simulink model "control_pid_nolineal"  (R2022b)
settings: Solver=ode45  StartTime=0.0  StopTime=30  MaxStep=0.01  RelTol=1e-3  EnableMultiTasking=on
values from neighbouring files (symbols this model uses):
  A = XX    [codigo_Prac5.m]
  k = As*sqrt(2*g)    [codigo_Prac5.m]
  Kp = XX    [codigo_Prac5.m]
  Q = 2    [codigo_Prac5.m]
  Td = XX    [codigo_Prac5.m]
  Ti = XX    [codigo_Prac5.m]
  x0_ini = [2*XX  XX]    [codigo_Prac5.m]
settings Model: Creator=carles  LastModifiedBy=ggarc
settings SolverCC: AlgebraicLoopSolver=TrustRegion
settings DataIOCC: LimitDataPoints=on  SaveFormat=Array  SignalLoggingSaveFormat=ModelDataLogs  ReturnWorkspaceOutputs=off
settings OptimizationCC: ExpressionDepthLimit=2147483647  LifeSpan=inf
settings DebuggingCC: UnderspecifiedInitializationDetection=Classic  MergeDetectMultiDrivingBlocksExec=none  SolverPrmCheckMsg=warning  FcnCallInpInsideContextMsg=warning  UnconnectedInputMsg=warning  UnconnectedOutputMsg=warning  UnconnectedLineMsg=warning  StateNameClashWarn=warning  SFUnexpectedBacktrackingDiag=warning  SFNoUnconditionalDefaultTransitionDiag=warning  SFExecutionAtInitializationDiag=none  SFMachineParentedDataDiag=warning  ArithmeticOperatorsInVariantConditions=warning
settings HardwareCC: ProdBitPerPointer=32  ProdBitPerSizeT=32  ProdBitPerPtrDiffT=32  ProdLargestAtomicFloat=None  ProdIntDivRoundTo=Undefined  ProdEndianess=Unspecified  ProdWordSize=32  ProdHWDeviceType=32-bit Generic
settings ModelReferenceCC: PropagateSignalLabelsOutOfModel=off
settings SFSimCC: SimUseLocalCustomCode=off  CustomCodeUndefinedFunction=UseInterfaceOnly
settings RTWCC: RTWUseLocalCustomCode=off
settings CodeAppCC: StateflowObjectComments=on
settings GRTTargetCC: TargetLangStandard=C89/C90 (ANSI)  CombineOutputUpdateFcns=off  GRTInterface=on
settings ConfigComp: CovMetricSettings=dw  CovSaveCumulativeToWorkspaceVar=on  CovSaveSingleToWorkspaceVar=on  CovExternalEMLEnable=off  CovSFcnEnable=off

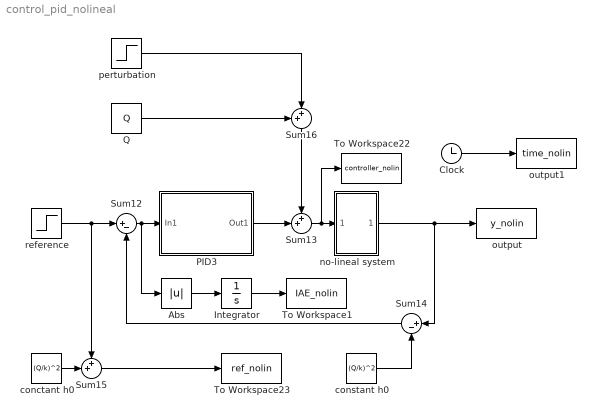
== system control_pid_nolineal ==
  Abs : Abs  SaturateOnIntegerOverflow=off
  Clock : Clock
  Integrator : Integrator
  PID3 : Subsystem
  Q : Constant  Value=Q
  Sum12 : Sum  Inputs=|+-
  Sum13 : Sum  Inputs=++|
  Sum14 : Sum  Inputs=|+-
  Sum15 : Sum  Inputs=++|
  Sum16 : Sum  Inputs=++|
  To Workspace1 : ToWorkspace  VariableName=IAE_nolin  SampleTime=-1
  To Workspace22 : ToWorkspace  VariableName=controller_nolin  SaveFormat=Structure With Time  SampleTime=-1
  To Workspace23 : ToWorkspace  VariableName=ref_nolin  SaveFormat=Structure With Time  SampleTime=-1
  conctant h0 : Constant  Value=(Q/k)^2
  constant h0 : Constant  Value=(Q/k)^2
  no-lineal system : Subsystem
  output : ToWorkspace  VariableName=y_nolin  SaveFormat=Structure With Time  SampleTime=-1
  output1 : ToWorkspace  VariableName=time_nolin  SampleTime=-1
  perturbation : Step  Time=30  After=2  SampleTime=0
  reference : Step  Time=5  After=0.2  SampleTime=0
  wires:
  Clock/1 -> output1/1
  Abs/1 -> Integrator/1
  Integrator/1 -> To Workspace1/1
  constant h0/1 -> Sum14/2
  Sum14/1 -> Sum12/2
  Sum12/1 -> Abs/1, PID3/1(In1)
  PID3/1(Out1) -> Sum13/2
  Sum13/1 -> To Workspace22/1, no-lineal system/1(In1)
  no-lineal system/1(Out2) -> output/1, Sum14/1
  reference/1 -> Sum12/1, Sum15/1
  conctant h0/1 -> Sum15/2
  Sum15/1 -> To Workspace23/1
  Sum16/1 -> Sum13/1
  Q/1 -> Sum16/1
  perturbation/1 -> Sum16/2

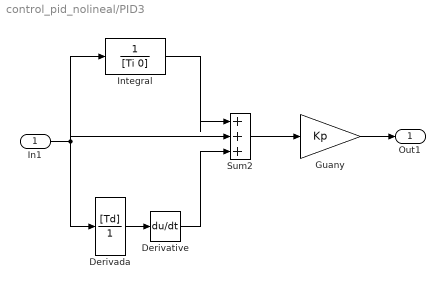
== system control_pid_nolineal/PID3 ==
  In1 : Inport
  Derivada : TransferFcn  Numerator=[Td]  Denominator=[1]
  Derivative : Derivative
  Guany : Gain  Gain=Kp
  Integral : TransferFcn  Denominator=[Ti 0]
  Sum2 : Sum  Inputs=|+++
  Out1 : Outport
  wires:
  Derivative/1 -> Sum2/3
  Derivada/1 -> Derivative/1
  In1/1 -> Integral/1, Derivada/1, Sum2/2
  Integral/1 -> Sum2/1
  Sum2/1 -> Guany/1
  Guany/1 -> Out1/1

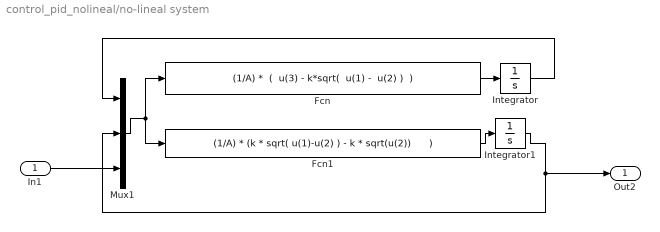
== system control_pid_nolineal/no-lineal system ==
  In1 : Inport
  Fcn : Fcn  Expr="(1/A) *  (  u(3) - k*sqrt(  u(1) -  u(2) )  )"
  Fcn1 : Fcn  Expr="(1/A) * (k * sqrt( u(1)-u(2) ) - k * sqrt(u(2))      )"
  Integrator : Integrator  InitialCondition=x0_ini(1)
  Integrator1 : Integrator  InitialCondition=x0_ini(2)
  Mux1 : Mux  Inputs=3
  Out2 : Outport
  wires:
  In1/1 -> Mux1/3
  Integrator1/1 -> Out2/1, Mux1/2
  Integrator/1 -> Mux1/1
  Mux1/1 -> Fcn/1, Fcn1/1
  Fcn1/1 -> Integrator1/1
  Fcn/1 -> Integrator/1
